simulink model "system1"  (R2023b)
settings: Solver=FixedStepAuto  StartTime=0.0  StopTime=Tmdl  FixedStep=Tmdl/n_steps  RelTol=1e-3
undefined symbols (not defined in the file): x1_initial, x2_initial
settings Model: Creator=deniskirbaba  LastModifiedBy=deniskirbaba

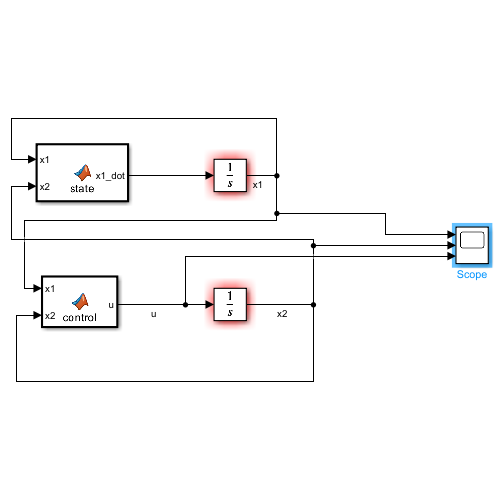
[thumbnail: Simulink's stored preview of the top-level diagram]
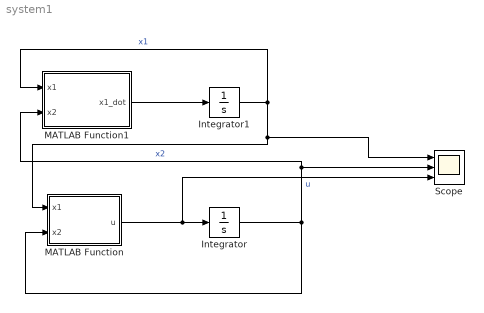
== system system1 ==
  Integrator : Integrator  InitialCondition=x2_initial
  Integrator1 : Integrator  InitialCondition=x1_initial
  MATLAB Function : MATLAB Function  TreatAsAtomicUnit=on
  MATLAB Function1 : MATLAB Function  TreatAsAtomicUnit=on
  Scope : Scope  NumInputPorts=3
  wires:
  Integrator/1 -> Scope/2, MATLAB Function1/2(x2), MATLAB Function/2(x2)  "x2"
  MATLAB Function1/1(x1_dot) -> Integrator1/1
  Integrator1/1 -> Scope/1, MATLAB Function/1(x1), MATLAB Function1/1(x1)  "x1"
  MATLAB Function/1(u) -> Scope/3, Integrator/1  "u"

== matlab function system1/MATLAB Function ==
  data: x1 input; u output; x2 input
function u = control(x1,x2)
z2 = x2+1.5*x1^2-x1;
u = -z2 + (-2*x1+1)*(-x1-0.5*x1^3-z2);

== matlab function system1/MATLAB Function1 ==
  data: x1 input; x1_dot output; x2 input
function x1_dot = state(x1,x2)

x1_dot = -x2-1.5*x1^2-0.5*x1^3;
